simulink model "thrust_vector_controlled_felix_nimy"  (R2024a)
settings: Solver=VariableStepAuto  StartTime=0.0  StopTime=125  RelTol=1e-3
libraries: simulink_extras x3, shared6dof x1, aerolibanim x1
settings Model: Creator=Felix NIMY  LastModifiedBy=Felix NIMY

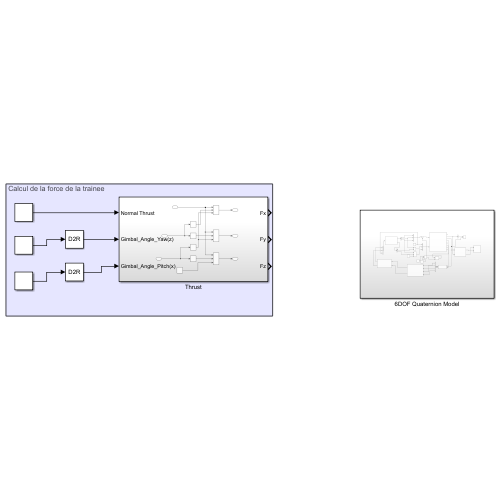
[thumbnail: Simulink's stored preview of the top-level diagram]
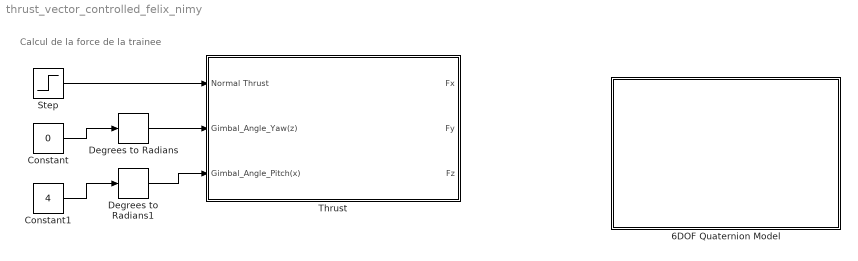
== system thrust_vector_controlled_felix_nimy ==
  note: Calcul de la force de la trainee
  6DOF Quaternion Model : Subsystem
  Constant : Constant  Value=0
  Constant1 : Constant  Value=4
  Degrees to Radians : simulink_extras/Transformations/Degrees to Radians
  Degrees to Radians1 : simulink_extras/Transformations/Degrees to Radians
  Step : Step  SampleTime=0
  Thrust : Subsystem
  wires:
  Step/1 -> Thrust/1(Normal Thrust)
  Constant/1 -> Degrees to Radians/1
  Degrees to Radians/1 -> Thrust/2(Gimbal_Angle_Yaw(z))
  Constant1/1 -> Degrees to Radians1/1
  Degrees to Radians1/1 -> Thrust/3(Gimbal_Angle_Pitch(x))

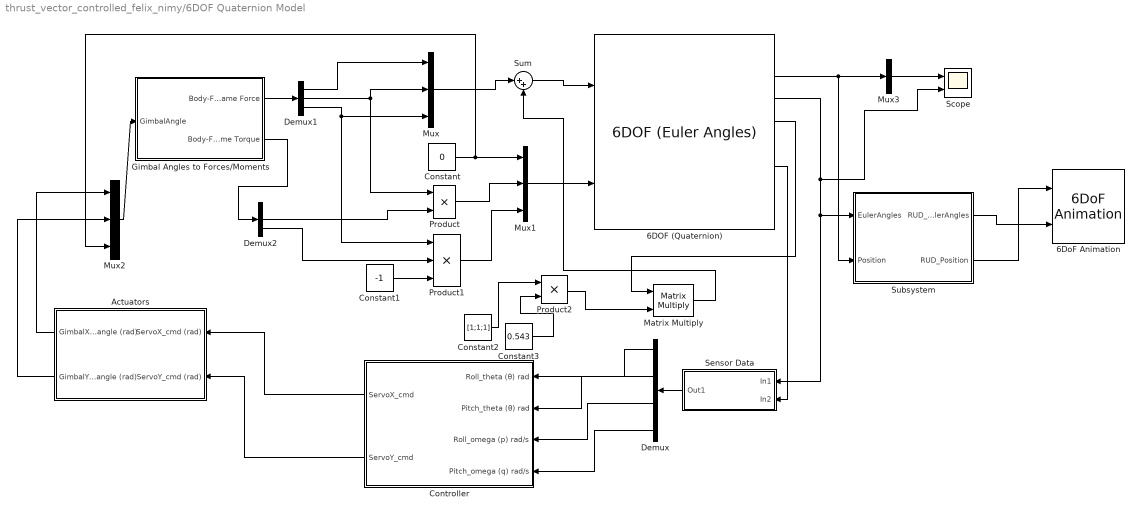
== system thrust_vector_controlled_felix_nimy/6DOF Quaternion Model ==
  6DOF (Quaternion) : shared6dof/6DOF (Euler Angles)  units=Metric (MKS)  mtype=Fixed  rep=Quaternion  xme_0=[0 0 0]  Vm_0=[0 0 0]  eul_0=[0 0 0]  pm_0=[0 0 0]  mass_0=1.0  mass_e=0.5  mass_f=2.0  inertia=eye(3)  inertia_e=eye(3)  inertia_f=2*eye(3)  k_quat=1.0  vre_flag=on  abi_flag=off  aMode=0  xme_statename=''  Vm_statename=''  eul_statename=''  quat_statename=''  pm_statename=''  mass_statename=''
      settings: LibrarySourceBlock=aerolib6dof2/6DOF (Quaternion)
  6DoF Animation : aerolibanim/6DoF Animation  u1=[0 4000 -2000 2000 -5000 -3000]  u2=0.1  u3=1.0  u4=[4000 0 -5000]  u5=Fixed position  u6=[2000 500 -3150]  u7=10  u8=on
  Actuators : Subsystem
  Constant : Constant  Value=0
  Constant1 : Constant  Value=-1
  Constant2 : Constant  Value=[1;1;1]
  Constant3 : Constant  Value=0.543
  Controller : Subsystem
  Demux : Demux
  Demux1 : Demux  Outputs=3
  Demux2 : Demux  Outputs=3
  Gimbal Angles to Forces/Moments : Subsystem
  Matrix Multiply : Product  Multiplication=Matrix(*)
  Mux : Mux  Inputs=3
  Mux1 : Mux  Inputs=3
  Mux2 : Mux  Inputs=3
  Mux3 : Mux  Inputs=1
  Product : Product
  Product1 : Product  Inputs=3
  Product2 : Product
  Scope : Scope  NumInputPorts=2
  Sensor Data : Subsystem
  Subsystem : Subsystem
  Sum : Sum  Inputs=|++
  wires:
  Mux/1 -> Sum/1
  Mux1/1 -> 6DOF (Quaternion)/2
  Constant/1 -> Mux2/3, Mux1/1
  Constant1/1 -> Product1/3
  Product/1 -> Mux1/2
  Product1/1 -> Mux1/3
  Constant3/1 -> Product2/2
  Constant2/1 -> Product2/1
  Product2/1 -> Matrix Multiply/2
  6DOF (Quaternion)/4 -> Matrix Multiply/1
  Matrix Multiply/1 -> Sum/2
  Sum/1 -> 6DOF (Quaternion)/1
  6DOF (Quaternion)/3 -> Sensor Data/1(In1), Subsystem/1(EulerAngles), Scope/2
  6DOF (Quaternion)/6 -> Sensor Data/2(In2)
  Sensor Data/1(Out1) -> Demux/1
  Demux/1 -> Controller/1(Roll_theta (θ) rad)
  Demux/2 -> Controller/2(Pitch_theta (θ) rad)
  Demux/3 -> Controller/3(Roll_omega (p) rad/s)
  Demux/4 -> Controller/4(Pitch_omega (q) rad/s)
  Controller/1(ServoX_cmd) -> Actuators/1(ServoX_cmd (rad))
  Controller/2(ServoY_cmd) -> Actuators/2(ServoY_cmd (rad))
  Mux2/1 -> Gimbal Angles to Forces/Moments/1(GimbalAngle)
  Actuators/1(GimbalX_angle (rad)) -> Mux2/1
  Actuators/2(GimbalY_angle (rad)) -> Mux2/2
  Gimbal Angles to Forces/Moments/1(Body-Frame Force) -> Demux1/1
  Demux1/1 -> Mux/1
  Demux1/3 -> Product1/1, Mux/3
  Demux1/2 -> Product/1, Mux/2
  Gimbal Angles to Forces/Moments/2(Body-Frame Torque) -> Demux2/1
  Demux2/2 -> Product/2
  Demux2/3 -> Product1/2
  Mux3/1 -> Scope/1
  6DOF (Quaternion)/2 -> Subsystem/2(Position), Mux3/1
  Subsystem/2(RUD_Position) -> 6DoF Animation/1
  Subsystem/1(RUD_EulerAngles) -> 6DoF Animation/2

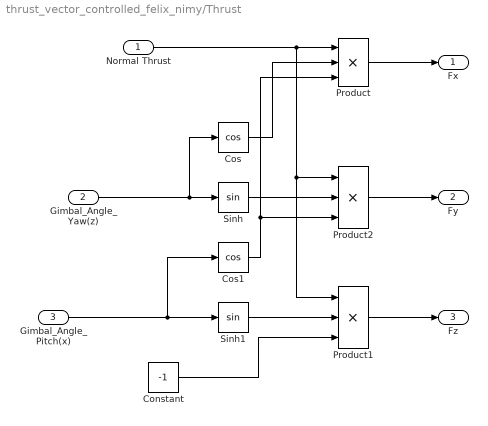
== system thrust_vector_controlled_felix_nimy/Thrust ==
  Normal Thrust : Inport
  Gimbal_Angle_Yaw(z) : Inport  Port=2
  Gimbal_Angle_Pitch(x) : Inport  Port=3
  Constant : Constant  Value=-1
  Cos : Trigonometry  Operator=cos
  Cos1 : Trigonometry  Operator=cos
  Product : Product  Inputs=3
  Product1 : Product  Inputs=3
  Product2 : Product  Inputs=3
  Sinh : Trigonometry
  Sinh1 : Trigonometry
  Fx : Outport
  Fy : Outport  Port=2
  Fz : Outport  Port=3
  wires:
  Normal Thrust/1 -> Product1/1, Product2/1, Product/1
  Gimbal_Angle_Yaw(z)/1 -> Cos/1, Sinh/1
  Cos/1 -> Product/2
  Sinh/1 -> Product2/2
  Gimbal_Angle_Pitch(x)/1 -> Cos1/1, Sinh1/1
  Cos1/1 -> Product2/3, Product/3
  Sinh1/1 -> Product1/2
  Constant/1 -> Product1/3
  Product1/1 -> Fz/1
  Product2/1 -> Fy/1
  Product/1 -> Fx/1

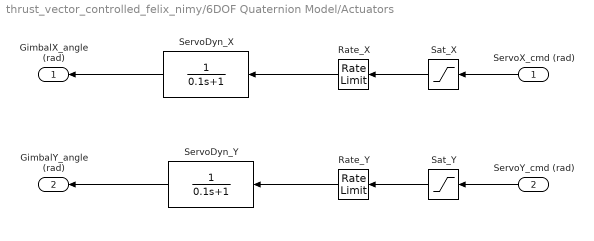
== system thrust_vector_controlled_felix_nimy/6DOF Quaternion Model/Actuators ==
  ServoX_cmd (rad) : Inport
  ServoY_cmd (rad) : Inport  Port=2
  Rate_X : RateLimiter  RisingSlewLimit=deg2rad(60)  FallingSlewLimit=-deg2rad(60)  SampleTimeMode=inherited
  Rate_Y : RateLimiter  RisingSlewLimit=deg2rad(60)  FallingSlewLimit=-deg2rad(60)  SampleTimeMode=inherited
  Sat_X : Saturate  UpperLimit=deg2rad(5)  LowerLimit=-deg2rad(5)
  Sat_Y : Saturate  UpperLimit=deg2rad(5)  LowerLimit=-deg2rad(5)
  ServoDyn_X : TransferFcn  Denominator=[0.1 1]
  ServoDyn_Y : TransferFcn  Denominator=[0.1 1]
  GimbalX_angle (rad) : Outport
  GimbalY_angle (rad) : Outport  Port=2
  wires:
  ServoX_cmd (rad)/1 -> Sat_X/1
  Rate_X/1 -> ServoDyn_X/1
  Rate_Y/1 -> ServoDyn_Y/1
  ServoDyn_Y/1 -> GimbalY_angle (rad)/1
  ServoDyn_X/1 -> GimbalX_angle (rad)/1
  Sat_X/1 -> Rate_X/1
  Sat_Y/1 -> Rate_Y/1
  ServoY_cmd (rad)/1 -> Sat_Y/1

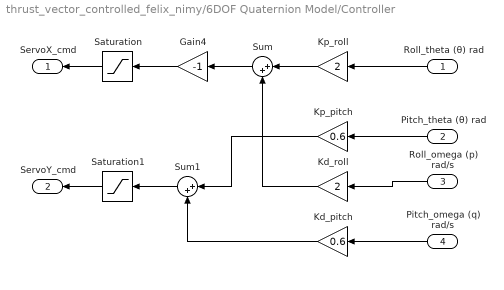
== system thrust_vector_controlled_felix_nimy/6DOF Quaternion Model/Controller ==
  Roll_theta (θ) rad : Inport
  Pitch_theta (θ) rad : Inport  Port=2
  Roll_omega (p) rad/s : Inport  Port=3
  Pitch_omega (q) rad/s : Inport  Port=4
  Gain4 : Gain  Gain=-1
  Kd_pitch : Gain  Gain=0.6
  Kd_roll : Gain  Gain=2
  Kp_pitch : Gain  Gain=0.6
  Kp_roll : Gain  Gain=2
  Saturation : Saturate  UpperLimit=deg2rad(5)  LowerLimit=-deg2rad(5)
  Saturation1 : Saturate  UpperLimit=deg2rad(5)  LowerLimit=-deg2rad(5)
  Sum : Sum  Inputs=|++
  Sum1 : Sum  Inputs=|++
  ServoX_cmd : Outport
  ServoY_cmd : Outport  Port=2
  wires:
  Roll_theta (θ) rad/1 -> Kp_roll/1
  Pitch_theta (θ) rad/1 -> Kp_pitch/1
  Roll_omega (p) rad/s/1 -> Kd_roll/1
  Pitch_omega (q) rad/s/1 -> Kd_pitch/1
  Kp_roll/1 -> Sum/1
  Kd_roll/1 -> Sum/2
  Sum/1 -> Gain4/1
  Kp_pitch/1 -> Sum1/1
  Kd_pitch/1 -> Sum1/2
  Gain4/1 -> Saturation/1
  Saturation/1 -> ServoX_cmd/1
  Sum1/1 -> Saturation1/1
  Saturation1/1 -> ServoY_cmd/1

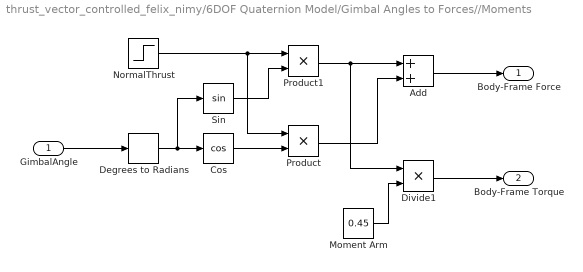
== system thrust_vector_controlled_felix_nimy/6DOF Quaternion Model/Gimbal Angles to Forces//Moments ==
  GimbalAngle : Inport
  Add : Sum
  Cos : Trigonometry  Operator=cos
  Degrees to Radians : simulink_extras/Transformations/Degrees to Radians
  Divide1 : Product  Inputs=**
  "Moment Arm " : Constant  Value=0.45
  NormalThrust : Step  Time=20  Before=15  After=0  SampleTime=0
  Product : Product  RndMeth=Zero
  Product1 : Product  RndMeth=Zero
  Sin : Trigonometry
  Body-Frame Force : Outport
  Body-Frame Torque : Outport  Port=2
  wires:
  Cos/1 -> Product/2
  NormalThrust/1 -> Product/1, Product1/1
  Sin/1 -> Product1/2
  Product1/1 -> Divide1/1, Add/1
  GimbalAngle/1 -> Degrees to Radians/1
  Degrees to Radians/1 -> Sin/1, Cos/1
  "Moment Arm "/1 -> Divide1/2
  Divide1/1 -> Body-Frame Torque/1
  Product/1 -> Add/2
  Add/1 -> Body-Frame Force/1

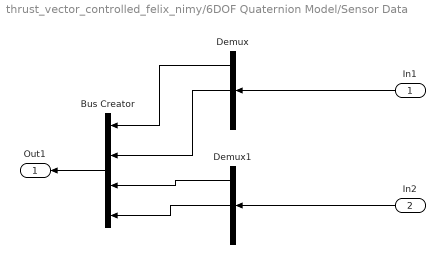
== system thrust_vector_controlled_felix_nimy/6DOF Quaternion Model/Sensor Data ==
  In1 : Inport
  In2 : Inport  Port=2
  Bus Creator : BusCreator  Inputs=4
  Demux : Demux  Outputs=3
  Demux1 : Demux  Outputs=3
  Out1 : Outport
  wires:
  In1/1 -> Demux/1
  In2/1 -> Demux1/1
  Demux/1 -> Bus Creator/1
  Demux/2 -> Bus Creator/2
  Demux1/1 -> Bus Creator/3
  Demux1/2 -> Bus Creator/4
  Bus Creator/1 -> Out1/1

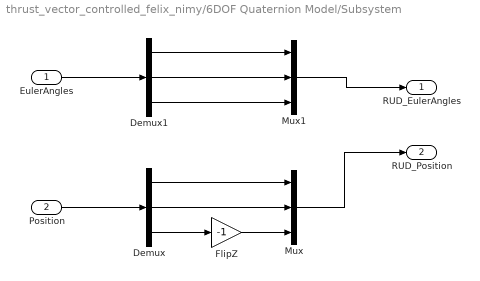
== system thrust_vector_controlled_felix_nimy/6DOF Quaternion Model/Subsystem ==
  EulerAngles : Inport
  Position : Inport  Port=2
  Demux : Demux  Outputs=3
  Demux1 : Demux  Outputs=3
  FlipZ : Gain  Gain=-1
  Mux : Mux  Inputs=3
  Mux1 : Mux  Inputs=3
  RUD_EulerAngles : Outport
  RUD_Position : Outport  Port=2
  wires:
  Position/1 -> Demux/1
  Demux/3 -> FlipZ/1
  FlipZ/1 -> Mux/3
  Demux/2 -> Mux/2
  Demux/1 -> Mux/1
  Mux/1 -> RUD_Position/1
  Mux1/1 -> RUD_EulerAngles/1
  Demux1/1 -> Mux1/1
  Demux1/2 -> Mux1/2
  Demux1/3 -> Mux1/3
  EulerAngles/1 -> Demux1/1
